simulink model "chapter_7"  (R2018b)
settings: Solver=VariableStepAuto  StartTime=0.0  StopTime=5  RelTol=1e-3
values from neighbouring files (symbols this model uses):
  c_sp = eye(2)    [FindF16Dynamics.m]
  K = place(a_sp, b_sp, [-2.743-4.75102i,-2.743+4.75102i])    [FindF16Dynamics.m]
undefined symbols (not defined in the file or in its folder): a_sp, b_sp, d_sp
settings Model: Creator=Marcel  LastModifiedBy=Marcel

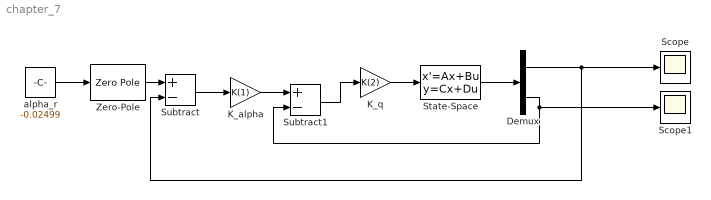
== system chapter_7 ==
  Demux : Demux  Outputs=2
  K_alpha : Gain  Gain=K(1)
  K_q : Gain  Gain=K(2)
  Scope : Scope
  Scope1 : Scope
  State-Space : StateSpace  A=a_sp  B=b_sp  C=c_sp  D=d_sp  InitialCondition=[0,0]
  Subtract : Sum  Inputs=+-
  Subtract1 : Sum  Inputs=+-
  Zero-Pole : ZeroPole  Zeros=[0.2340]  Poles=[-0.8749]
  alpha_r : Constant  Value=-0.02499
  wires:
  State-Space/1 -> Demux/1
  alpha_r/1 -> Zero-Pole/1
  Demux/1 -> Scope/1, Subtract/2
  Subtract/1 -> K_alpha/1
  K_alpha/1 -> Subtract1/1
  Demux/2 -> Subtract1/2, Scope1/1
  K_q/1 -> State-Space/1
  Subtract1/1 -> K_q/1
  Zero-Pole/1 -> Subtract/1
